simulink model "adapt_model"  (R2013a)
settings: Solver=ode45  StartTime=0.0  StopTime=50  RelTol=1e-3
values from neighbouring files (symbols this model uses):
  A = [S3 S6 S7;S6 S8 S9; S7 S9 S10]    [LSQ_regression.m]
undefined symbols (not defined in the file or in its folder): C
settings Model: Creator=Aleksandr  LastModifiedBy=Aleksandr

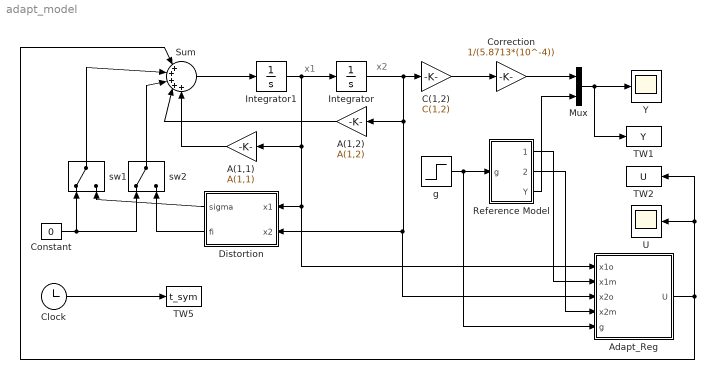
== system adapt_model ==
  note: x2
  note: x1
  A(1,1) : Gain  Gain=A(1,1)
  A(1,2) : Gain  Gain=A(1,2)
  Adapt_Reg : Subsystem
  C(1,2) : Gain  Gain=C(1,2)
  Clock : Clock
      settings: Decimation=2000
  Constant : Constant  Value=0
  Correction : Gain  Gain=1/(5.8713*(10^-4))
  Distortion : Subsystem
  Integrator : Integrator
  Integrator1 : Integrator
  Mux : Mux  Inputs=2
  Reference Model : Subsystem
  Sum : Sum  Inputs=|+++++
  TW1 : ToWorkspace  VariableName=Y  SampleTime=-1
  TW2 : ToWorkspace  VariableName=U  SampleTime=-1
  TW5 : ToWorkspace  VariableName=t_sym  SampleTime=-1
  U : Scope
      settings: TimeRange=2000  YMin=0  YMax=1  SaveName=ScopeData3
  Y : Scope
      settings: TimeRange=66.00660066006603  YMin=0.1940823327615782  YMax=0.2156946826758149
  g : Step  Time=0  SampleTime=0
  sw1 : ManualSwitch
  sw2 : ManualSwitch
  wires:
  Integrator1/1 -> Integrator/1, Distortion/1(x1), Adapt_Reg/1(x1o), A(1,1)/1
  Integrator/1 -> C(1,2)/1, Adapt_Reg/3(x2o), Distortion/2(x2), A(1,2)/1
  Mux/1 -> TW1/1, Y/1
  A(1,1)/1 -> Sum/5
  A(1,2)/1 -> Sum/4
  Distortion/1(sigma) -> sw1/2
  Distortion/2(fi) -> sw2/2
  sw2/1 -> Sum/3
  sw1/1 -> Sum/2
  Reference Model/3(Y) -> Mux/2
  Reference Model/1(x1m) -> Adapt_Reg/2(x1m)
  Reference Model/2(x2m) -> Adapt_Reg/4(x2m)
  Constant/1 -> sw2/1, sw1/1
  Clock/1 -> TW5/1
  Sum/1 -> Integrator1/1
  Adapt_Reg/1(U) -> TW2/1, U/1, Sum/1
  C(1,2)/1 -> Correction/1
  Correction/1 -> Mux/1
  g/1 -> Adapt_Reg/5(g), Reference Model/1(g)

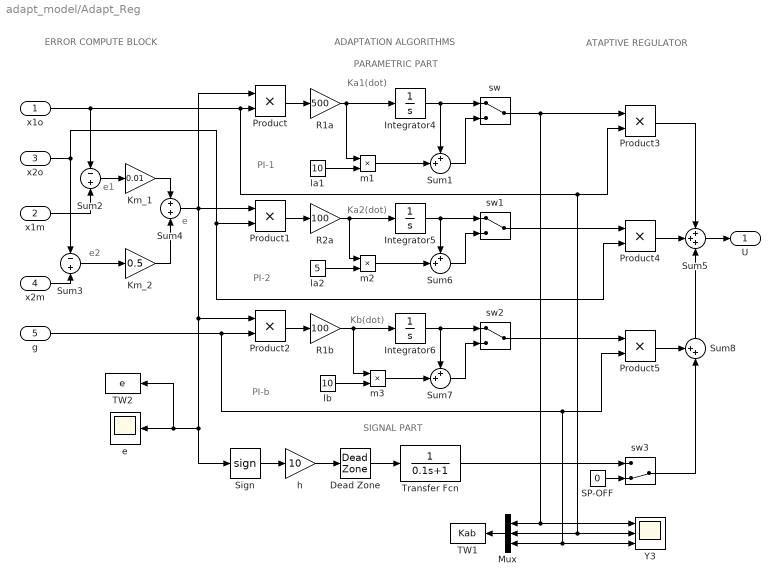
== system adapt_model/Adapt_Reg ==
  note: PARAMETRIC PART
  note: SIGNAL PART
  note: PI-b
  note: PI-2
  note: PI-1
  note: ATAPTIVE REGULATOR
  note: ADAPTATION ALGORITHMS
  note: ERROR COMPUTE BLOCK
  note: Ka1(dot)
  note: e
  note: e2
  note: e1
  note: Ka2(dot)
  note: Kb(dot)
  x1o : Inport
  x1m : Inport  Port=2
  x2o : Inport  Port=3
  x2m : Inport  Port=4
  g : Inport  Port=5
  Dead Zone : DeadZone  SaturateOnIntegerOverflow=on
  Integrator4 : Integrator
  Integrator5 : Integrator
  Integrator6 : Integrator
  Km_1 : Gain  Gain=0.01
  Km_2 : Gain  Gain=0.5
  Mux : Mux  Inputs=3
  Product{,1..5} (6 alike) : Product
  R1a : Gain  Gain=500
  R1b : Gain  Gain=100
  R2a : Gain  Gain=100
  SP-OFF : Constant  Value=0
  Sign : Signum  ZeroCross=off
  Sum{1,6..8} (4 alike) : Sum  Inputs=++|
  Sum2 : Sum  Inputs=-+
  Sum3 : Sum  Inputs=-+
  Sum4 : Sum
  Sum5 : Sum  Inputs=+++
  TW1 : ToWorkspace  VariableName=Kab  SampleTime=-1
  TW2 : ToWorkspace  VariableName=e  SampleTime=-1
  Transfer Fcn : TransferFcn  Denominator=[0.1 1]
  Y3 : Scope  NumInputPorts=3
      settings: TimeRange=2000  YMin=0~-5~-5  YMax=1~5~5
  e : Scope
      settings: TimeRange=2000  YMin=0  YMax=1  SaveName=ScopeData2
  h : Gain  Gain=10
  la1 : Constant  Value=10
  la2 : Constant  Value=5
  lb : Constant  Value=10
  m1 : Product
  m2 : Product
  m3 : Product
  sw : ManualSwitch
  sw1 : ManualSwitch
  sw2 : ManualSwitch
  sw3 : ManualSwitch  CurrentSetting=0
  U : Outport
  wires:
  Km_2/1 -> Sum4/2
  Sum3/1 -> Km_2/1
  Km_1/1 -> Sum4/1
  x2o/1 -> Product1/2, Product4/2, Sum3/1
  x2m/1 -> Sum3/2
  Product2/1 -> R1b/1
  Product1/1 -> R2a/1
  x1o/1 -> Y3/2, Mux/2, Product3/2, Product/2, Sum2/1
  Sum2/1 -> Km_1/1
  Product/1 -> R1a/1
  Integrator5/1 -> sw1/1, Sum6/1
  Integrator4/1 -> sw/1, Sum1/1
  Sum5/1 -> U/1
  R2a/1 -> m2/1, Integrator5/1
  Product3/1 -> Sum5/1
  x1m/1 -> Sum2/2
  Product4/1 -> Sum5/2
  R1a/1 -> m1/1, Integrator4/1
  g/1 -> Y3/3, Mux/3, Product5/2, Product2/2
  la1/1 -> m1/2
  m1/1 -> Sum1/2
  Sum1/1 -> sw/2
  la2/1 -> m2/2
  m2/1 -> Sum6/2
  Sum6/1 -> sw1/2
  Integrator6/1 -> sw2/1, Sum7/1
  R1b/1 -> Integrator6/1, m3/1
  lb/1 -> m3/2
  m3/1 -> Sum7/2
  Sum7/1 -> sw2/2
  Sign/1 -> h/1
  h/1 -> Dead Zone/1
  Dead Zone/1 -> Transfer Fcn/1
  Sum8/1 -> Sum5/3
  Product5/1 -> Sum8/1
  Transfer Fcn/1 -> sw3/1
  sw3/1 -> Sum8/2
  SP-OFF/1 -> sw3/2
  sw/1 -> Mux/1, Y3/1, Product3/1
  sw1/1 -> Product4/1
  sw2/1 -> Product5/1
  Sum4/1 -> TW2/1, e/1, Sign/1, Product2/1, Product/1, Product1/1
  Mux/1 -> TW1/1

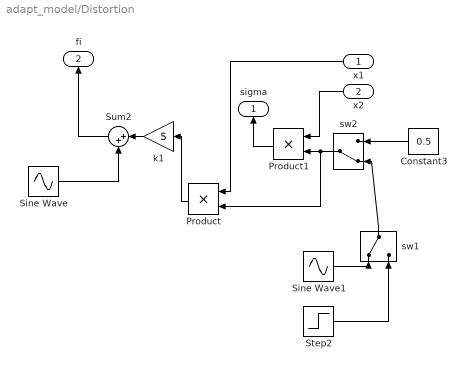
== system adapt_model/Distortion ==
  x1 : Inport
  x2 : Inport  Port=2
  Constant3 : Constant  Value=0.5
  Product : Product
  Product1 : Product
  Sine Wave : Sin  Amplitude=5  Frequency=pi/2  SampleTime=0
  Sine Wave1 : Sin  SampleTime=0
  Step2 : Step  Time=0  After=2.5  SampleTime=0
  Sum2 : Sum  Inputs=|++
  k1 : Gain  Gain=5
  sw1 : ManualSwitch
  sw2 : ManualSwitch  CurrentSetting=0
  sigma : Outport
  fi : Outport  Port=2
  wires:
  x1/1 -> Product/1
  Product1/1 -> sigma/1
  Sum2/1 -> fi/1
  Sine Wave1/1 -> sw1/1
  x2/1 -> Product1/1
  sw2/1 -> Product/2, Product1/2
  Step2/1 -> sw1/2
  Product/1 -> k1/1
  k1/1 -> Sum2/1
  Sine Wave/1 -> Sum2/2
  Constant3/1 -> sw2/1
  sw1/1 -> sw2/2

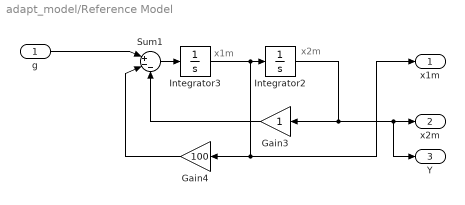
== system adapt_model/Reference Model ==
  note: x2m
  note: x1m
  g : Inport
  Gain3 : Gain
  Gain4 : Gain  Gain=100
  Integrator2 : Integrator
  Integrator3 : Integrator
  Sum1 : Sum  Inputs=|+--
  x1m : Outport
  x2m : Outport  Port=2
  Y : Outport  Port=3
  wires:
  Integrator2/1 -> Y/1, x2m/1, Gain3/1
  g/1 -> Sum1/1
  Sum1/1 -> Integrator3/1
  Gain4/1 -> Sum1/2
  Integrator3/1 -> Gain4/1, x1m/1, Integrator2/1
  Gain3/1 -> Sum1/3
